simulink model "new68bus_opal"  (R2019b)
settings: Solver=ode4  StartTime=0.0  StopTime=30  FixedStep=Ts  RelTol=1e-3
PreLoadFcn:
  | PSSMODEL=1;
  | LPSS=0;
  | WAPSS=0;
  | WAPSS2=0;
  | Ts=50e-5;
InitFcn:
  | PSSMODEL=1;
  | LPSS=0;
  | WAPSS=0;
  | WAPSS2=0;
  | Ts=50e-5;
  | 
  | % Required data to 68 Bus benchmark
  | % clear
  | % clc
  | % Definition for the columns
  | % system base =100 MVA
  | 
  | %% Line data Format (line)
  | % All values are given on the same system base MVA
  | % 1: From bus
  | % 2: To bus
  | % 3: Resistance (pu)
  | % 4: Reactance  (pu)
  | % 5: Charge     (pu)
  | % 6: Transformer Tap Amplitute
  | % 7: base MVA
  | % 8: Nomonal Voltage (KV)
  | 
  | %1   2    3        4       5       6        7      8
  | line=[...
  | 1	54	0	     0.0181	  0	      1.025     100    13.8
  | 2	58	0	     0.025	  0	      1.070     100    13.8
  | 3	62	0	     0.02	  0	      1.070     100    13.8
  | 4	19	0.0007	 0.0142	  0	      1.070     100    13.8
  | 5	20	0.0009	 0.018	  0	      1.009     100    13.8
  | 6	22	0	     0.0143	  0	      1.025     100    13.8
  | 7	23	0.0005	 0.0272	  0	      0         100    13.8
  | 8	25	0.0006	 0.0232	  0	      1.025     100    13.8
  | 9	29	0.0008	 0.0156   0	      1.025     100    13.8
  | 10	31	0	     0.026	  0	      1.04      100    13.8
  | 11	32	0	     0.013	  0	      1.04      100    13.8
  | 12	36	0	     0.0075	  0	      1.04      100    13.8
  | 13	17	0	     0.0033	  0	      1.04      100    13.8
  | 14	41	0	     0.0015	  0	      1         100    13.8
  | 15	42	0	     0.0015	  0	      1         100    13.8
  | 16	18	0	     0.003	  0	      1         100    13.8
  | 17	36	0.0005	 0.0045	  0.32	  0         100    138
  | 17	43	0.0005	 0.0276	  0	      0         100    138
  | 18	42	0.004	 0.06	  2.25    0         100    138
  | 18	49	0.0076	 0.1141	  1.16    0	        100    138
  | 18	50	0.0012	 0.0288	  2.06	  0         100    138
  | 20	19	0.0007	 0.0138	  0       1.06	    100    138
  | 19	68	0.0016	 0.0195	  0.304	  0         100    138
  | 21	22	0.0008	 0.014	  0.2565  0	        100    138
  | 21	68	0.0008	 0.0135	  0.2548  0	        100    138
  | 22	23	0.0006	 0.0096	  0.1846  0	        100    138
  | 23	24	0.0022	 0.035	  0.361	  0         100    138
  | 24	68	0.0003	 0.0059	  0.068	  0         100    138
  | 25	26	0.0032	 0.0323	  0.531	  0         100    138
  | 25	54	0.007	 0.0086	  0.146	  0         100    138
  | 26	27	0.0014	 0.0147	  0.2396  0	        100    138
  | 26	28	0.0043	 0.0474	  0.7802  0	        100    138
  | 26	29	0.0057	 0.0625	  1.029	  0         100    138
  | 27	37	0.0013	 0.0173	  0.3216  0	        100    138
  | 27	53	0.032	 0.32	  0.41	  0         100    138
  | ... (+206 lines)
undefined symbols (not defined in the file or in its folder): D1, Delta, I, Left, Right, type, V
libraries: powerlib x359, artemis x26, sps_avr x16, powerlib_meascontrol x5, rtlab x1
(part 3 of 8)

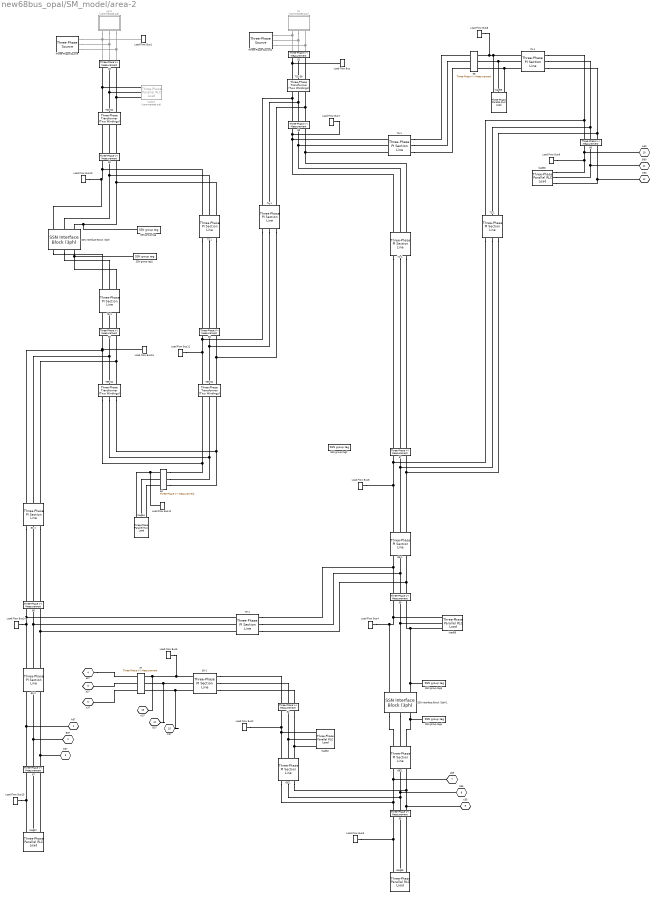
== system new68bus_opal/SM_model/area-2 ==
  02 : powerlib/Measurements/Three-Phase V-I Measurement  VoltageMeasurement=phase-to-phase  SetLabelV=on  LabelV=Vabc_02  Vpu=off  VpuLL=on  CurrentMeasurement=no  SetLabelI=off  LabelI=Iabc  Ipu=off  Pbase=100e6  Vbase=13.8e3  OutputType=Complex  PhasorSimulation=off  PSBequivalent=0
      settings: SourceProductName=Simscape Electrical
  03 : powerlib/Measurements/Three-Phase V-I Measurement  VoltageMeasurement=phase-to-phase  SetLabelV=on  LabelV=Vabc_03  Vpu=off  VpuLL=on  CurrentMeasurement=no  SetLabelI=off  LabelI=Iabc  Ipu=off  Pbase=100e6  Vbase=13.8e3  OutputType=Complex  PhasorSimulation=off  PSBequivalent=0
      settings: SourceProductName=Simscape Electrical
  37 : powerlib/Measurements/Three-Phase V-I Measurement  VoltageMeasurement=phase-to-phase  SetLabelV=on  LabelV=Vabc_37  Vpu=off  VpuLL=on  CurrentMeasurement=no  SetLabelI=off  LabelI=Iabc  Ipu=off  Pbase=100e6  Vbase=Bus(37,2)*1e3  OutputType=Complex  PhasorSimulation=off  PSBequivalent=0
      settings: SourceProductName=Simscape Electrical
  50-1 : powerlib/Elements/Three-Phase PI Section Line  LConnTagsString=a|b|c  RConnTagsString=A|B|C  Frequency=60  Resistances=[line(50,3) 3*line(50,3)]  Inductances=[line(50,4) 3*line(50,4)]  Capacitances=[line(50,5) line(50,5)/3]  Length=1
      settings: SourceProductName=Simscape Electrical
  52 : powerlib/Measurements/Three-Phase V-I Measurement  VoltageMeasurement=phase-to-phase  SetLabelV=on  LabelV=Vabc_52  Vpu=off  VpuLL=on  CurrentMeasurement=no  SetLabelI=off  LabelI=Iabc  Ipu=off  Pbase=100e6  Vbase=Bus(52,2)*1e3  OutputType=Complex  PhasorSimulation=off  PSBequivalent=0
      settings: SourceProductName=Simscape Electrical
  55 : powerlib/Measurements/Three-Phase V-I Measurement  VoltageMeasurement=phase-to-phase  SetLabelV=on  LabelV=Vabc_55  Vpu=off  VpuLL=on  CurrentMeasurement=no  SetLabelI=off  LabelI=Iabc  Ipu=off  Pbase=100e6  Vbase=Bus(55,2)*1e3  OutputType=Complex  PhasorSimulation=off  PSBequivalent=0
      settings: SourceProductName=Simscape Electrical
  56 : powerlib/Measurements/Three-Phase V-I Measurement  VoltageMeasurement=phase-to-phase  SetLabelV=on  LabelV=Vabc_56  Vpu=off  VpuLL=on  CurrentMeasurement=no  SetLabelI=off  LabelI=Iabc  Ipu=off  Pbase=100e6  Vbase=Bus(56,2)*1e3  OutputType=Complex  PhasorSimulation=off  PSBequivalent=0
      settings: SourceProductName=Simscape Electrical
  57 : powerlib/Measurements/Three-Phase V-I Measurement  VoltageMeasurement=phase-to-phase  SetLabelV=on  LabelV=Vabc_57  Vpu=off  VpuLL=on  CurrentMeasurement=no  SetLabelI=off  LabelI=Iabc  Ipu=off  Pbase=100e6  Vbase=Bus(57,2)*1e3  OutputType=Complex  PhasorSimulation=off  PSBequivalent=0
      settings: SourceProductName=Simscape Electrical
  58 : powerlib/Measurements/Three-Phase V-I Measurement  VoltageMeasurement=phase-to-phase  SetLabelV=on  LabelV=Vabc_58  Vpu=off  VpuLL=on  CurrentMeasurement=no  SetLabelI=off  LabelI=Iabc  Ipu=off  Pbase=100e6  Vbase=Bus(58,2)*1e3  OutputType=Complex  PhasorSimulation=off  PSBequivalent=0
      settings: SourceProductName=Simscape Electrical
  59 : powerlib/Measurements/Three-Phase V-I Measurement  VoltageMeasurement=phase-to-phase  SetLabelV=on  LabelV=Vabc_59  Vpu=off  VpuLL=on  CurrentMeasurement=no  SetLabelI=off  LabelI=Iabc  Ipu=off  Pbase=100e6  Vbase=Bus(59,2)*1e3  OutputType=Complex  PhasorSimulation=off  PSBequivalent=0
      settings: SourceProductName=Simscape Electrical
  60 : powerlib/Measurements/Three-Phase V-I Measurement  VoltageMeasurement=phase-to-phase  SetLabelV=on  LabelV=Vabc_60  Vpu=off  VpuLL=on  CurrentMeasurement=no  SetLabelI=off  LabelI=Iabc  Ipu=off  Pbase=100e6  Vbase=Bus(60,2)*1e3  OutputType=Complex  PhasorSimulation=off  PSBequivalent=0
      settings: SourceProductName=Simscape Electrical
  62 : powerlib/Measurements/Three-Phase V-I Measurement  VoltageMeasurement=phase-to-phase  SetLabelV=on  LabelV=Vabc_62  Vpu=off  VpuLL=on  CurrentMeasurement=no  SetLabelI=off  LabelI=Iabc  Ipu=off  Pbase=100e6  Vbase=Bus(62,2)*1e3  OutputType=Complex  PhasorSimulation=off  PSBequivalent=0
      settings: SourceProductName=Simscape Electrical
  63 : powerlib/Measurements/Three-Phase V-I Measurement  VoltageMeasurement=phase-to-phase  SetLabelV=on  LabelV=Vabc_63  Vpu=off  VpuLL=on  CurrentMeasurement=no  SetLabelI=off  LabelI=Iabc  Ipu=off  Pbase=100e6  Vbase=Bus(63,2)*1e3  OutputType=Complex  PhasorSimulation=off  PSBequivalent=0
      settings: SourceProductName=Simscape Electrical
  64 : powerlib/Measurements/Three-Phase V-I Measurement  VoltageMeasurement=phase-to-phase  SetLabelV=on  LabelV=Vabc_64  Vpu=off  VpuLL=on  CurrentMeasurement=no  SetLabelI=off  LabelI=Iabc  Ipu=off  Pbase=100e6  Vbase=Bus(64,2)*1e3  OutputType=Complex  PhasorSimulation=off  PSBequivalent=0
      settings: SourceProductName=Simscape Electrical
  65 : powerlib/Measurements/Three-Phase V-I Measurement  VoltageMeasurement=phase-to-phase  SetLabelV=on  LabelV=Vabc_65  Vpu=off  VpuLL=on  CurrentMeasurement=no  SetLabelI=off  LabelI=Iabc  Ipu=off  Pbase=100e6  Vbase=Bus(65,2)*1e3  OutputType=Complex  PhasorSimulation=off  PSBequivalent=0
      settings: SourceProductName=Simscape Electrical
  65-1 : powerlib/Elements/Three-Phase PI Section Line  LConnTagsString=a|b|c  RConnTagsString=A|B|C  Frequency=60  Resistances=[line(65,3) 3*line(65,3)]  Inductances=[line(65,4) 3*line(65,4)]  Capacitances=[line(65,5) line(65,5)/3]  Length=1
      settings: SourceProductName=Simscape Electrical
  66 : powerlib/Measurements/Three-Phase V-I Measurement  VoltageMeasurement=phase-to-phase  SetLabelV=on  LabelV=Vabc_66  Vpu=off  VpuLL=on  CurrentMeasurement=no  SetLabelI=off  LabelI=Iabc  Ipu=off  Pbase=100e6  Vbase=Bus(66,2)*1e3  OutputType=Complex  PhasorSimulation=off  PSBequivalent=0
      settings: SourceProductName=Simscape Electrical
  67 : powerlib/Measurements/Three-Phase V-I Measurement  VoltageMeasurement=phase-to-phase  SetLabelV=on  LabelV=Vabc_67  Vpu=off  VpuLL=on  CurrentMeasurement=no  SetLabelI=off  LabelI=Iabc  Ipu=off  Pbase=100e6  Vbase=Bus(67,2)*1e3  OutputType=Complex  PhasorSimulation=off  PSBequivalent=0
      settings: SourceProductName=Simscape Electrical
  68-1 : powerlib/Elements/Three-Phase PI Section Line  LConnTagsString=a|b|c  RConnTagsString=A|B|C  Frequency=60  Resistances=[line(68,3) 3*line(68,3)]  Inductances=[line(68,4) 3*line(68,4)]  Capacitances=[line(68,5) line(68,5)/3]  Length=1
      settings: SourceProductName=Simscape Electrical
  69-1 : powerlib/Elements/Three-Phase PI Section Line  LConnTagsString=a|b|c  RConnTagsString=A|B|C  Frequency=60  Resistances=[line(69,3) 3*line(69,3)]  Inductances=[line(69,4) 3*line(69,4)]  Capacitances=[line(69,5) line(69,5)/3]  Length=1
      settings: SourceProductName=Simscape Electrical
  70-1 : powerlib/Elements/Three-Phase PI Section Line  LConnTagsString=a|b|c  RConnTagsString=A|B|C  Frequency=60  Resistances=[line(70,3) 3*line(70,3)]  Inductances=[line(70,4) 3*line(70,4)]  Capacitances=[line(70,5) line(70,5)/3]  Length=1
      settings: SourceProductName=Simscape Electrical
  71-1 : powerlib/Elements/Three-Phase PI Section Line  LConnTagsString=a|b|c  RConnTagsString=A|B|C  Frequency=60  Resistances=[line(71,3) 3*line(71,3)]  Inductances=[line(71,4) 3*line(71,4)]  Capacitances=[line(71,5) line(71,5)/3]  Length=1
      settings: SourceProductName=Simscape Electrical
  72-1 : powerlib/Elements/Three-Phase PI Section Line  LConnTagsString=a|b|c  RConnTagsString=A|B|C  Frequency=60  Resistances=[line(72,3) 3*line(72,3)]  Inductances=[line(72,4) 3*line(72,4)]  Capacitances=[line(72,5) line(72,5)/3]  Length=1
      settings: SourceProductName=Simscape Electrical
  73-1 : powerlib/Elements/Three-Phase PI Section Line  LConnTagsString=a|b|c  RConnTagsString=A|B|C  Frequency=60  Resistances=[line(73,3) 3*line(73,3)]  Inductances=[line(73,4) 3*line(73,4)]  Capacitances=[line(73,5) line(73,5)/3]  Length=1
      settings: SourceProductName=Simscape Electrical
  74-1 : powerlib/Elements/Three-Phase PI Section Line  LConnTagsString=a|b|c  RConnTagsString=A|B|C  Frequency=60  Resistances=[line(74,3) 3*line(74,3)]  Inductances=[line(74,4) 3*line(74,4)]  Capacitances=[line(74,5) line(74,5)/3]  Length=1
      settings: SourceProductName=Simscape Electrical
  75-1 : powerlib/Elements/Three-Phase PI Section Line  LConnTagsString=a|b|c  RConnTagsString=A|B|C  Frequency=60  Resistances=[line(75,3) 3*line(75,3)]  Inductances=[line(75,4) 3*line(75,4)]  Capacitances=[line(75,5) line(75,5)/3]  Length=1
      settings: SourceProductName=Simscape Electrical
  77-1 : powerlib/Elements/Three-Phase PI Section Line  LConnTagsString=a|b|c  RConnTagsString=A|B|C  Frequency=60  Resistances=[line(77,3) 3*line(77,3)]  Inductances=[line(77,4) 3*line(77,4)]  Capacitances=[line(77,5) line(77,5)/3]  Length=1
      settings: SourceProductName=Simscape Electrical
  78-1 : powerlib/Elements/Three-Phase PI Section Line  LConnTagsString=a|b|c  RConnTagsString=A|B|C  Frequency=60  Resistances=[line(78,3) 3*line(78,3)]  Inductances=[line(78,4) 3*line(78,4)]  Capacitances=[line(78,5) line(78,5)/3]  Length=1
      settings: SourceProductName=Simscape Electrical
  81-1 : powerlib/Elements/Three-Phase PI Section Line  LConnTagsString=a|b|c  RConnTagsString=A|B|C  Frequency=60  Resistances=[line(81,3) 3*line(81,3)]  Inductances=[line(81,4) 3*line(81,4)]  Capacitances=[line(81,5) line(81,5)/3]  Length=1
      settings: SourceProductName=Simscape Electrical
  81-2 : powerlib/Elements/Three-Phase PI Section Line  LConnTagsString=a|b|c  RConnTagsString=A|B|C  Frequency=60  Resistances=[line(81,3) 3*line(81,3)]  Inductances=[line(81,4) 3*line(81,4)]  Capacitances=[line(81,5) line(81,5)/3]  Length=1
      settings: SourceProductName=Simscape Electrical
  G2 : Subsystem  Commented=on
  Load Flow Bus : powerlib/Measurements/Load Flow Bus  LConnTagsString=a  Phases=single  Connectors=on one side  ID=BUS_02  Vbase=13.8e3  Vref=0.98  Vangle=0  VLF=1  VLFb=1  VLFc=1  angleLF=0  angleLFb=0  angleLFc=0
      settings: SourceProductName=Simscape Electrical
  Load Flow Bus1 : powerlib/Measurements/Load Flow Bus  LConnTagsString=a  Phases=single  Connectors=on one side  ID=BUS_03  Vbase=13.8e3  Vref=0.983  Vangle=0  VLF=1  VLFb=1  VLFc=1  angleLF=0  angleLFb=0  angleLFc=0
      settings: SourceProductName=Simscape Electrical
  Load Flow Bus10 : powerlib/Measurements/Load Flow Bus  LConnTagsString=a  Phases=single  Connectors=on one side  ID=BUS_62  Vbase=138e3  Vref=1  Vangle=0  VLF=1  VLFb=1  VLFc=1  angleLF=0  angleLFb=0  angleLFc=0
      settings: SourceProductName=Simscape Electrical
  Load Flow Bus11 : powerlib/Measurements/Load Flow Bus  LConnTagsString=a  Phases=single  Connectors=on one side  ID=BUS_63  Vbase=138e3  Vref=1  Vangle=0  VLF=1  VLFb=1  VLFc=1  angleLF=0  angleLFb=0  angleLFc=0
      settings: SourceProductName=Simscape Electrical
  Load Flow Bus12 : powerlib/Measurements/Load Flow Bus  LConnTagsString=a  Phases=single  Connectors=on one side  ID=BUS_64  Vbase=138e3  Vref=1  Vangle=0  VLF=1  VLFb=1  VLFc=1  angleLF=0  angleLFb=0  angleLFc=0
      settings: SourceProductName=Simscape Electrical
  Load Flow Bus13 : powerlib/Measurements/Load Flow Bus  LConnTagsString=a  Phases=single  Connectors=on one side  ID=BUS_65  Vbase=138e3  Vref=1  Vangle=0  VLF=1  VLFb=1  VLFc=1  angleLF=0  angleLFb=0  angleLFc=0
      settings: SourceProductName=Simscape Electrical
  Load Flow Bus14 : powerlib/Measurements/Load Flow Bus  LConnTagsString=a  Phases=single  Connectors=on one side  ID=BUS_66  Vbase=138e3  Vref=1  Vangle=0  VLF=1  VLFb=1  VLFc=1  angleLF=0  angleLFb=0  angleLFc=0
      settings: SourceProductName=Simscape Electrical
  Load Flow Bus15 : powerlib/Measurements/Load Flow Bus  LConnTagsString=a  Phases=single  Connectors=on one side  ID=BUS_67  Vbase=138e3  Vref=1  Vangle=0  VLF=1  VLFb=1  VLFc=1  angleLF=0  angleLFb=0  angleLFc=0
      settings: SourceProductName=Simscape Electrical
  Load Flow Bus2 : powerlib/Measurements/Load Flow Bus  LConnTagsString=a  Phases=single  Connectors=on one side  ID=BUS_52  Vbase=138e3  Vref=1  Vangle=0  VLF=1  VLFb=1  VLFc=1  angleLF=0  angleLFb=0  angleLFc=0
      settings: SourceProductName=Simscape Electrical
  Load Flow Bus3 : powerlib/Measurements/Load Flow Bus  LConnTagsString=a  Phases=single  Connectors=on one side  ID=BUS_55  Vbase=138e3  Vref=1  Vangle=0  VLF=1  VLFb=1  VLFc=1  angleLF=0  angleLFb=0  angleLFc=0
      settings: SourceProductName=Simscape Electrical
  Load Flow Bus4 : powerlib/Measurements/Load Flow Bus  LConnTagsString=a  Phases=single  Connectors=on one side  ID=BUS_56  Vbase=138e3  Vref=1  Vangle=0  VLF=1  VLFb=1  VLFc=1  angleLF=0  angleLFb=0  angleLFc=0
      settings: SourceProductName=Simscape Electrical
  Load Flow Bus5 : powerlib/Measurements/Load Flow Bus  LConnTagsString=a  Phases=single  Connectors=on one side  ID=BUS_37  Vbase=138e3  Vref=1  Vangle=0  VLF=1  VLFb=1  VLFc=1  angleLF=0  angleLFb=0  angleLFc=0
      settings: SourceProductName=Simscape Electrical
  Load Flow Bus6 : powerlib/Measurements/Load Flow Bus  LConnTagsString=a  Phases=single  Connectors=on one side  ID=BUS_57  Vbase=138e3  Vref=1  Vangle=0  VLF=1  VLFb=1  VLFc=1  angleLF=0  angleLFb=0  angleLFc=0
      settings: SourceProductName=Simscape Electrical
  Load Flow Bus7 : powerlib/Measurements/Load Flow Bus  LConnTagsString=a  Phases=single  Connectors=on one side  ID=BUS_58  Vbase=138e3  Vref=1  Vangle=0  VLF=1  VLFb=1  VLFc=1  angleLF=0  angleLFb=0  angleLFc=0
      settings: SourceProductName=Simscape Electrical
  Load Flow Bus8 : powerlib/Measurements/Load Flow Bus  LConnTagsString=a  Phases=single  Connectors=on one side  ID=BUS_59  Vbase=138e3  Vref=1  Vangle=0  VLF=1  VLFb=1  VLFc=1  angleLF=0  angleLFb=0  angleLFc=0
      settings: SourceProductName=Simscape Electrical
  Load Flow Bus9 : powerlib/Measurements/Load Flow Bus  LConnTagsString=a  Phases=single  Connectors=on one side  ID=BUS_60  Vbase=138e3  Vref=1  Vangle=0  VLF=1  VLFb=1  VLFc=1  angleLF=0  angleLFb=0  angleLFc=0
      settings: SourceProductName=Simscape Electrical
  SSN Interface Block (3ph) : artemis/SSN/Nodal Interface Blocks/SSN Interface Block (3ph)  nb_phase=3  nb_port=2  p1_type=I-type(Left)  p2_type=I-type(Right)  p3_type=V-type(Left)  p4_type=V-type(Left)  p5_type=V-type(Left)  p6_type=V-type(Left)  p7_type=V-type(Left)  p8_type=V-type(Left)  p9_type=V-type(Left)  p10_type=V-type(Left)  p11_type=V-type(Left)  p12_type=V-type(Left)  p13_type=V-type(Left)  p14_type=V-type(Left)  p15_type=V-type(Left)  p16_type=V-type(Left)  I_port_shunt_resistance=1e9
  SSN Interface Block (3ph)1 : artemis/SSN/Nodal Interface Blocks/SSN Interface Block (3ph)  nb_phase=3  nb_port=2  p1_type=I-type(Left)  p2_type=I-type(Right)  p3_type=V-type(Left)  p4_type=V-type(Left)  p5_type=V-type(Left)  p6_type=V-type(Left)  p7_type=V-type(Left)  p8_type=V-type(Left)  p9_type=V-type(Left)  p10_type=V-type(Left)  p11_type=V-type(Left)  p12_type=V-type(Left)  p13_type=V-type(Left)  p14_type=V-type(Left)  p15_type=V-type(Left)  p16_type=V-type(Left)  I_port_shunt_resistance=1e9
  SSN group tag : artemis/SSN/SSN group tag  ssn_group_tag=ssn5a
  SSN group tag1 : artemis/SSN/SSN group tag  ssn_group_tag=ssn5b
  SSN group tag2 : artemis/SSN/SSN group tag  ssn_group_tag=ssn5a
  SSN group tag3 : artemis/SSN/SSN group tag  ssn_group_tag=ssn6a
  SSN group tag4 : artemis/SSN/SSN group tag  ssn_group_tag=ssn6b
  T02-58 : powerlib/Elements/Three-Phase Transformer (Two Windings)  Winding1Connection=Delta (D1)  Winding2Connection=Yg  CoreType=Three single-phase transformers  SetSaturation=off  Hysteresis=off  DataFile='hysteresis'  SetInitialFlux=off  Measurements=None  UNITS=pu  NominalPower=[ 10000e6 , 60 ]  Winding1=[ 13.8e3 , 0.0002 , 0 ]  Winding2=[ 138e3 , 0 .0002, 0.0125]  Rm=500  Lm=500  L0=0.5  Saturation=[ 0,0 ; 0.0024,1.2 ; 1.0,1.52 ]  InitialFluxes=[ 0.8 , -0.8 , 0.7 ]  BreakLoop=off  DiscreteSolver=Trapezoidal robust  DataType=off  TransfoNumber=1
      settings: SourceProductName=Simscape Electrical
  T03-62 : powerlib/Elements/Three-Phase Transformer (Two Windings)  Winding1Connection=Delta (D1)  Winding2Connection=Yg  CoreType=Three single-phase transformers  SetSaturation=off  Hysteresis=off  DataFile='hysteresis'  SetInitialFlux=off  Measurements=None  UNITS=pu  NominalPower=[ 10000e6 , 60 ]  Winding1=[ 13.8e3 , 0.000 , 0 ]  Winding2=[ 138e3 , 0.000, 0.0101]  Rm=500  Lm=500  L0=0.5  Saturation=[ 0,0 ; 0.0024,1.2 ; 1.0,1.52 ]  InitialFluxes=[ 0.8 , -0.8 , 0.7 ]  BreakLoop=off  DiscreteSolver=Trapezoidal robust  DataType=off  TransfoNumber=1
      settings: SourceProductName=Simscape Electrical
  T63-64 : powerlib/Elements/Three-Phase Transformer (Two Windings)  Winding1Connection=Y  Winding2Connection=Y  CoreType=Three single-phase transformers  SetSaturation=off  Hysteresis=off  DataFile='hysteresis'  SetInitialFlux=off  Measurements=None  UNITS=pu  NominalPower=[ 10000e6 , 60 ]  Winding1=[ 138e3 , 0.152, 0 ]  Winding2=[ 138e3 , 0.152 , 0.022]  Rm=500  Lm=500  L0=0.5  Saturation=[ 0,0 ; 0.0024,1.2 ; 1.0,1.52 ]  InitialFluxes=[ 0.8 , -0.8 , 0.7 ]  BreakLoop=off  DiscreteSolver=Trapezoidal robust  DataType=off  TransfoNumber=1
      settings: SourceProductName=Simscape Electrical
  T65-64 : powerlib/Elements/Three-Phase Transformer (Two Windings)  Winding1Connection=Y  Winding2Connection=Y  CoreType=Three single-phase transformers  SetSaturation=off  Hysteresis=off  DataFile='hysteresis'  SetInitialFlux=off  Measurements=None  UNITS=pu  NominalPower=[ 10000e6 , 60 ]  Winding1=[ 138e3 , 0.152, 0 ]  Winding2=[ 138e3 , 0.152 , 0.022]  Rm=500  Lm=500  L0=0.5  Saturation=[ 0,0 ; 0.0024,1.2 ; 1.0,1.52 ]  InitialFluxes=[ 0.8 , -0.8 , 0.7 ]  BreakLoop=off  DiscreteSolver=Trapezoidal robust  DataType=off  TransfoNumber=1
      settings: SourceProductName=Simscape Electrical
  Three-Phase Source : powerlib/Electrical Sources/Three-Phase Source  InternalConnection=Yg  VoltagePhases=off  Voltage=13.8e3  PhaseAngle=0  Voltage_phases=[25e3 25e3 25e3]/sqrt(3)  PhaseAngles_phases=[0 -120 +120]  Frequency=60  NonIdealSource=on  SpecifyImpedance=off  Resistance=0.8929  Inductance=16.58e-3  ShortCircuitLevel=100e6  BaseVoltage=13.8e3  XRratio=7  BusType=PV  Pref=650e6  Qref=0  Prefabc=[10e3, 10e3, 10e3]  Qrefabc=[0, 0, 0]  Qmin=-inf  Qmax=inf
      settings: SourceProductName=Simscape Electrical
  Three-Phase Source1 : powerlib/Electrical Sources/Three-Phase Source  InternalConnection=Yg  VoltagePhases=off  Voltage=13.8e3  PhaseAngle=0  Voltage_phases=[25e3 25e3 25e3]/sqrt(3)  PhaseAngles_phases=[0 -120 +120]  Frequency=60  NonIdealSource=on  SpecifyImpedance=off  Resistance=0.8929  Inductance=16.58e-3  ShortCircuitLevel=100e6  BaseVoltage=13.8e3  XRratio=7  BusType=PV  Pref=545e6  Qref=0  Prefabc=[10e3, 10e3, 10e3]  Qrefabc=[0, 0, 0]  Qmin=-inf  Qmax=inf
      settings: SourceProductName=Simscape Electrical
  gen3 : Subsystem  Commented=on
  load03 : powerlib/Elements/Three-Phase Parallel RLC Load  Commented=on  LConnTagsString=A|B|C  Configuration=Y (grounded)  NominalVoltage=138000  Vabc=[1e3 1e3 1e3]  Vabcp=[1e3 1e3 1e3]  NominalFrequency=60  UnbalancedPower=off  ActivePower=0  InductivePower=50e06  CapacitivePower=0  Pabc=[10e3 9e3 11e3]  QLabc=[100 90 110]  QCabc=[100 90 110]  Pabcp=[10e3 9e3 11e3]  QLabcp=[100 90 110]  QCabcp=[100 90 110]  Measurements=None  LoadType=constant PQ
      settings: SourceProductName=Simscape Electrical
  load52 : powerlib/Elements/Three-Phase Parallel RLC Load  LConnTagsString=A|B|C  Configuration=Y (grounded)  NominalVoltage=138000  Vabc=[1e3 1e3 1e3]  Vabcp=[1e3 1e3 1e3]  NominalFrequency=60  UnbalancedPower=off  ActivePower=158e06  InductivePower=30e06  CapacitivePower=0  Pabc=[10e3 9e3 11e3]  QLabc=[100 90 110]  QCabc=[100 90 110]  Pabcp=[10e3 9e3 11e3]  QLabcp=[100 90 110]  QCabcp=[100 90 110]  Measurements=None  LoadType=constant PQ
      settings: SourceProductName=Simscape Electrical
  load55 : powerlib/Elements/Three-Phase Parallel RLC Load  LConnTagsString=A|B|C  Configuration=Y (grounded)  NominalVoltage=138000  Vabc=[1e3 1e3 1e3]  Vabcp=[1e3 1e3 1e3]  NominalFrequency=60  UnbalancedPower=off  ActivePower=322e06  InductivePower=2e06  CapacitivePower=0  Pabc=[10e3 9e3 11e3]  QLabc=[100 90 110]  QCabc=[100 90 110]  Pabcp=[10e3 9e3 11e3]  QLabcp=[100 90 110]  QCabcp=[100 90 110]  Measurements=None  LoadType=constant PQ
      settings: SourceProductName=Simscape Electrical
  load56 : powerlib/Elements/Three-Phase Parallel RLC Load  LConnTagsString=A|B|C  Configuration=Y (grounded)  NominalVoltage=138000  Vabc=[1e3 1e3 1e3]  Vabcp=[1e3 1e3 1e3]  NominalFrequency=60  UnbalancedPower=off  ActivePower=200e06  InductivePower=74e06  CapacitivePower=0  Pabc=[10e3 9e3 11e3]  QLabc=[100 90 110]  QCabc=[100 90 110]  Pabcp=[10e3 9e3 11e3]  QLabcp=[100 90 110]  QCabcp=[100 90 110]  Measurements=None  LoadType=constant PQ
      settings: SourceProductName=Simscape Electrical
  load59 : powerlib/Elements/Three-Phase Parallel RLC Load  LConnTagsString=A|B|C  Configuration=Y (grounded)  NominalVoltage=138000  Vabc=[1e3 1e3 1e3]  Vabcp=[1e3 1e3 1e3]  NominalFrequency=60  UnbalancedPower=off  ActivePower=234e06  InductivePower=84e06  CapacitivePower=0  Pabc=[10e3 9e3 11e3]  QLabc=[100 90 110]  QCabc=[100 90 110]  Pabcp=[10e3 9e3 11e3]  QLabcp=[100 90 110]  QCabcp=[100 90 110]  Measurements=None  LoadType=constant PQ
      settings: SourceProductName=Simscape Electrical
  load60 : powerlib/Elements/Three-Phase Parallel RLC Load  LConnTagsString=A|B|C  Configuration=Y (grounded)  NominalVoltage=138000  Vabc=[1e3 1e3 1e3]  Vabcp=[1e3 1e3 1e3]  NominalFrequency=60  UnbalancedPower=off  ActivePower=209e06  InductivePower=71e06  CapacitivePower=0  Pabc=[10e3 9e3 11e3]  QLabc=[100 90 110]  QCabc=[100 90 110]  Pabcp=[10e3 9e3 11e3]  QLabcp=[100 90 110]  QCabcp=[100 90 110]  Measurements=None  LoadType=constant PQ
      settings: SourceProductName=Simscape Electrical
  load64 : powerlib/Elements/Three-Phase Parallel RLC Load  LConnTagsString=A|B|C  Configuration=Y (grounded)  NominalVoltage=138000  Vabc=[1e3 1e3 1e3]  Vabcp=[1e3 1e3 1e3]  NominalFrequency=60  UnbalancedPower=off  ActivePower=9e06  InductivePower=88e06  CapacitivePower=0  Pabc=[10e3 9e3 11e3]  QLabc=[100 90 110]  QCabc=[100 90 110]  Pabcp=[10e3 9e3 11e3]  QLabcp=[100 90 110]  QCabcp=[100 90 110]  Measurements=None  LoadType=constant PQ
      settings: SourceProductName=Simscape Electrical
  load67 : powerlib/Elements/Three-Phase Parallel RLC Load  LConnTagsString=A|B|C  Configuration=Y (grounded)  NominalVoltage=138000  Vabc=[1e3 1e3 1e3]  Vabcp=[1e3 1e3 1e3]  NominalFrequency=60  UnbalancedPower=off  ActivePower=320e06  InductivePower=153e06  CapacitivePower=0  Pabc=[10e3 9e3 11e3]  QLabc=[100 90 110]  QCabc=[100 90 110]  Pabcp=[10e3 9e3 11e3]  QLabcp=[100 90 110]  QCabcp=[100 90 110]  Measurements=None  LoadType=constant PQ
      settings: SourceProductName=Simscape Electrical
  A67 : PMIOPort  Tag=PMCPort  Side=Right
  B67 : PMIOPort  Tag=PMCPort  Port=2  Side=Right
  C67 : PMIOPort  Tag=PMCPort  Port=3  Side=Right
  a37 : PMIOPort  Tag=PMCPort  Port=4  Side=Right
  c37 : PMIOPort  Tag=PMCPort  Port=5  Side=Right
  b37 : PMIOPort  Tag=PMCPort  Port=6  Side=Right
  a55 : PMIOPort  Tag=PMCPort  Port=7  Side=Right
  b55 : PMIOPort  Tag=PMCPort  Port=8  Side=Right
  c55 : PMIOPort  Tag=PMCPort  Port=9  Side=Right
  A60 : PMIOPort  Tag=PMCPort  Port=10  Side=Right
  B60 : PMIOPort  Tag=PMCPort  Port=11  Side=Right
  C60 : PMIOPort  Tag=PMCPort  Port=12  Side=Right
  A37 : PMIOPort  Tag=PMCPort  Port=13  Side=Right
  B37 : PMIOPort  Tag=PMCPort  Port=14  Side=Right
  C37 : PMIOPort  Tag=PMCPort  Port=15  Side=Right
  connections:
  gen3/LConn2 -- Three-Phase Source/RConn2 -- 03/RConn2
  62/RConn3 -- T03-62/RConn3
  T03-62/LConn1 -- 03/LConn1 -- load03/LConn1
  T03-62/LConn2 -- 03/LConn2 -- load03/LConn2
  62/RConn2 -- T03-62/RConn2
  62/RConn1 -- T03-62/RConn1
  gen3/LConn3 -- Three-Phase Source/RConn3 -- 03/RConn3
  gen3/LConn1 -- Load Flow Bus1/LConn1 -- Three-Phase Source/RConn1 -- 03/RConn1
  T03-62/LConn3 -- 03/LConn3 -- load03/LConn3
  Load Flow Bus10/LConn1 -- SSN Interface Block (3ph)/LConn1 -- 77-1/RConn1 -- 62/LConn1
  77-1/RConn2 -- SSN Interface Block (3ph)/LConn2 -- 62/LConn2
  77-1/RConn3 -- SSN group tag/LConn1 -- SSN Interface Block (3ph)/LConn3 -- 62/LConn3
  65/RConn1 -- 78-1/LConn1
  65/RConn2 -- 78-1/LConn2
  65/RConn3 -- 78-1/LConn3
  77-1/LConn1 -- 63/RConn1
  77-1/LConn2 -- 63/RConn2
  77-1/LConn3 -- 63/RConn3
  T63-64/LConn1 -- Load Flow Bus11/LConn1 -- 63/LConn1 -- 74-1/RConn1
  63/LConn2 -- T63-64/LConn2 -- 74-1/RConn2
  63/LConn3 -- T63-64/LConn3 -- 74-1/RConn3
  64/RConn1 -- T63-64/RConn1 -- T65-64/RConn1
  T63-64/RConn2 -- 64/RConn2 -- T65-64/RConn2
  T63-64/RConn3 -- 64/RConn3 -- T65-64/RConn3
  T65-64/LConn1 -- Load Flow Bus13/LConn1 -- 65/LConn1 -- 81-1/RConn1
  T65-64/LConn2 -- 81-1/RConn2 -- 65/LConn2
  T65-64/LConn3 -- 81-1/RConn3 -- 65/LConn3
  load64/LConn1 -- Load Flow Bus12/LConn1 -- 64/LConn1
  load64/LConn2 -- 64/LConn2
  load64/LConn3 -- 64/LConn3
  81-1/LConn1 -- 66/RConn1
  81-1/LConn2 -- 66/RConn2
  81-1/LConn3 -- 66/RConn3
  81-2/RConn1 -- Load Flow Bus14/LConn1 -- 66/LConn1 -- 70-1/RConn1
  81-2/RConn2 -- 66/LConn2 -- 70-1/RConn2
  81-2/RConn3 -- 66/LConn3 -- 70-1/RConn3
  81-2/LConn1 -- 67/RConn1 -- A67/RConn1
  67/RConn2 -- 81-2/LConn2 -- B67/RConn1
  C67/RConn1 -- 67/RConn3 -- 81-2/LConn3
  G2/LConn1 -- Three-Phase Source1/RConn1 -- 02/RConn1
  G2/LConn2 -- Three-Phase Source1/RConn2 -- 02/RConn2
  G2/LConn3 -- Three-Phase Source1/RConn3 -- 02/RConn3
  02/LConn1 -- T02-58/LConn1 -- Load Flow Bus/LConn1
  T02-58/LConn2 -- 02/LConn2
  T02-58/LConn3 -- 02/LConn3
  T02-58/RConn1 -- 58/RConn1 -- 74-1/LConn1
  T02-58/RConn2 -- 58/RConn2 -- 74-1/LConn2
  T02-58/RConn3 -- 58/RConn3 -- 74-1/LConn3
  73-1/RConn1 -- 71-1/RConn1 -- Load Flow Bus7/LConn1 -- 58/LConn1
  71-1/RConn2 -- 73-1/RConn2 -- 58/LConn2
  71-1/RConn3 -- 73-1/RConn3 -- 58/LConn3
  71-1/LConn1 -- 57/RConn1
  71-1/LConn2 -- 57/RConn2
  71-1/LConn3 -- 57/RConn3
  73-1/LConn1 -- 59/RConn1
  73-1/LConn2 -- 59/RConn2
  73-1/LConn3 -- 59/RConn3
  75-1/RConn1 -- load59/LConn1 -- Load Flow Bus8/LConn1 -- 59/LConn1
  75-1/RConn2 -- load59/LConn2 -- 59/LConn2
  75-1/RConn3 -- load59/LConn3 -- 59/LConn3
  75-1/LConn1 -- 60/RConn1 -- 72-1/LConn1
  75-1/LConn2 -- 60/RConn2 -- 72-1/LConn2
  75-1/LConn3 -- 60/RConn3 -- 72-1/LConn3
  A60/RConn1 -- load60/LConn1 -- Load Flow Bus9/LConn1 -- 60/LConn1
  load60/LConn2 -- 60/LConn2 -- B60/RConn1
  load60/LConn3 -- C60/RConn1 -- 60/LConn3
  69-1/RConn1 -- 57/LConn1 -- 72-1/RConn1 -- Load Flow Bus6/LConn1
  57/LConn2 -- 69-1/RConn2 -- 72-1/RConn2
  57/LConn3 -- 69-1/RConn3 -- 72-1/RConn3
  69-1/LConn1 -- 56/RConn1 -- 70-1/LConn1
  69-1/LConn2 -- 56/RConn2 -- 70-1/LConn2
  56/RConn3 -- 70-1/LConn3 -- 69-1/LConn3
  Load Flow Bus4/LConn1 -- load56/LConn1 -- 56/LConn1 -- SSN Interface Block (3ph)1/LConn1
  load56/LConn2 -- SSN Interface Block (3ph)1/LConn2 -- 56/LConn2
  load56/LConn3 -- SSN Interface Block (3ph)1/LConn3 -- SSN group tag3/LConn1 -- 56/LConn3
  68-1/LConn1 -- 55/RConn1 -- 65-1/LConn1 -- a55/RConn1
  b55/RConn1 -- 55/RConn2 -- 65-1/LConn2 -- 68-1/LConn2
  65-1/LConn3 -- 68-1/LConn3 -- 55/RConn3 -- c55/RConn1
  load67/LConn1 -- Load Flow Bus15/LConn1 -- 67/LConn1
  load67/LConn2 -- 67/LConn2
  load67/LConn3 -- 67/LConn3
  65-1/RConn1 -- 52/LConn1 -- Load Flow Bus2/LConn1 -- load52/LConn1
  65-1/RConn2 -- load52/LConn2 -- 52/LConn2
  65-1/RConn3 -- load52/LConn3 -- 52/LConn3
  load55/LConn1 -- Load Flow Bus3/LConn1 -- 55/LConn1
  load55/LConn2 -- 55/LConn2
  load55/LConn3 -- 55/LConn3
  a37/RConn1 -- 37/RConn1
  37/RConn2 -- b37/RConn1
  37/RConn3 -- c37/RConn1
  37/LConn1 -- Load Flow Bus5/LConn1 -- 50-1/RConn1 -- A37/RConn1
  50-1/RConn2 -- B37/RConn1 -- 37/LConn2
  37/LConn3 -- 50-1/RConn3 -- C37/RConn1
  50-1/LConn1 -- 52/RConn1
  50-1/LConn2 -- 52/RConn2
  50-1/LConn3 -- 52/RConn3
  SSN Interface Block (3ph)/RConn3 -- 78-1/RConn3 -- SSN group tag1/LConn1
  SSN Interface Block (3ph)/RConn2 -- 78-1/RConn2
  SSN Interface Block (3ph)/RConn1 -- 78-1/RConn1
  SSN Interface Block (3ph)1/RConn2 -- 68-1/RConn2
  SSN Interface Block (3ph)1/RConn1 -- 68-1/RConn1
  SSN Interface Block (3ph)1/RConn3 -- 68-1/RConn3 -- SSN group tag4/LConn1
